simulink model "Rocket_Simulation"  (R2024a)
settings: Solver=VariableStepAuto  StartTime=0.0  StopTime=25  RelTol=1e-3
values from neighbouring files (symbols this model uses):
  g = -9.80665    [OpenRocketDataLoader.m]
undefined symbols (not defined in the file or in its folder): magnitude
libraries: simulink x3, aerolibactuator x1, aerolibatmos2 x1
settings Model: Creator=bennettbabu  LastModifiedBy=mason

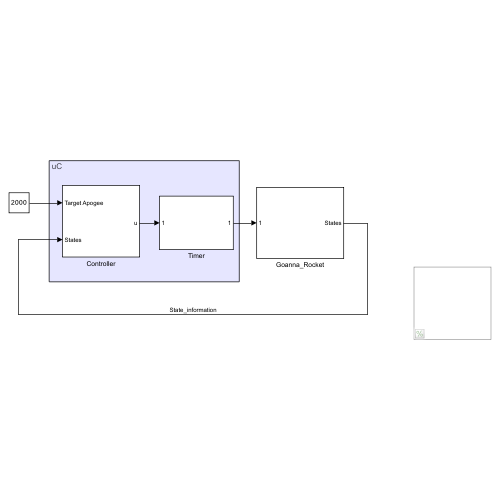
[thumbnail: Simulink's stored preview of the top-level diagram]
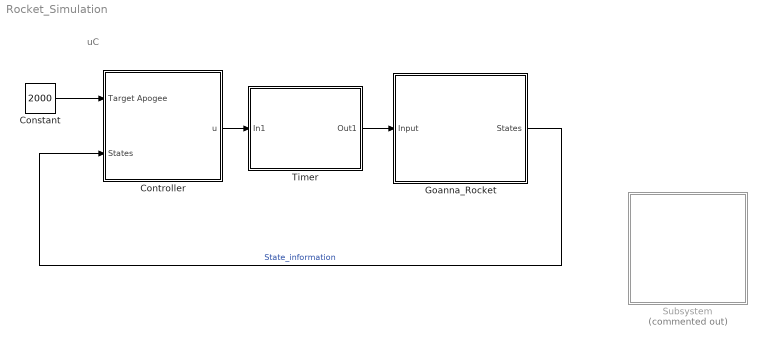
== system Rocket_Simulation ==
  note: uC
  Constant : Constant  Value=2000
  Controller : Subsystem
  Goanna_Rocket : Subsystem
  Subsystem : Subsystem  Commented=on
  Timer : Subsystem
  wires:
  Goanna_Rocket/1(States) -> Controller/2(States)  "State_information"
  Constant/1 -> Controller/1(Target Apogee)
  Controller/1(u) -> Timer/1(In1)
  Timer/1(Out1) -> Goanna_Rocket/1(Input)

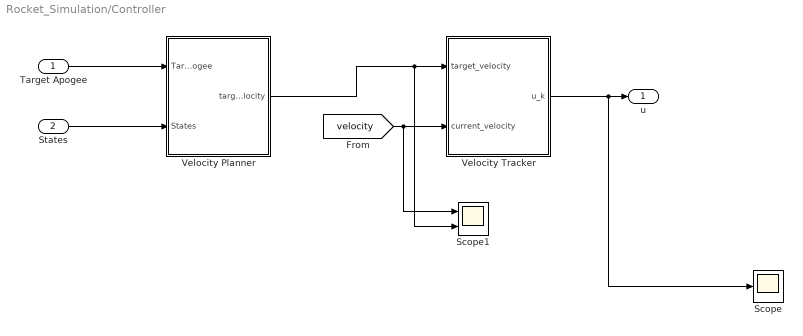
== system Rocket_Simulation/Controller ==
  Target Apogee : Inport
  States : Inport  Port=2
  Scope : Scope
  Scope1 : Scope  NumInputPorts=2
  Velocity Planner : Subsystem
  Velocity Tracker : Subsystem
  u : Outport
  wires:
  Target Apogee/1 -> Velocity Planner/1(Target Apogee)
  States/1 -> Velocity Planner/2(States)
  Velocity Tracker/1(u_k) -> Scope/1, u/1
  [velocity] -> Scope1/1, Velocity Tracker/2(current_velocity)
  Velocity Planner/1(target_velocity) -> Scope1/2, Velocity Tracker/1(target_velocity)

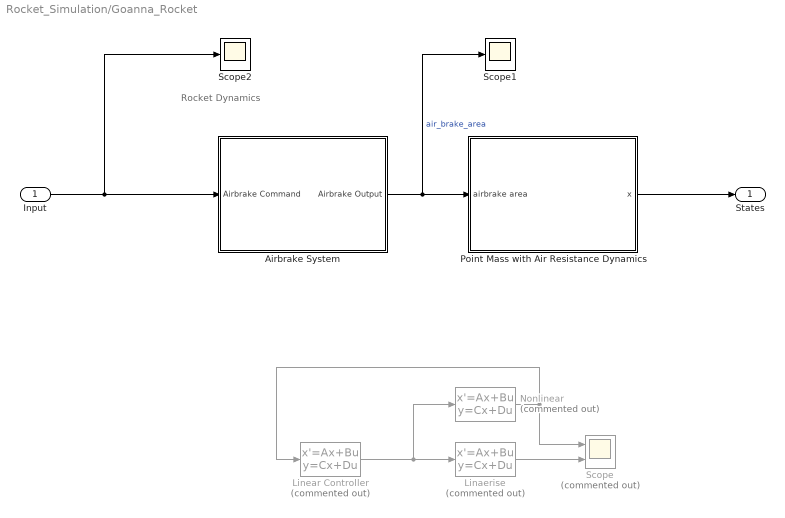
== system Rocket_Simulation/Goanna_Rocket ==
  note: Rocket Dynamics
  Input : Inport
  Airbrake System : Subsystem
      mask Display: image('airbrake.png');
  "Linaerise " : StateSpace  Commented=on  InitialCondition=0
  Linear Controller : StateSpace  Commented=on  InitialCondition=0
  Nonlinear : StateSpace  Commented=on  InitialCondition=0
  "Point Mass with Air Resistance Dynamics " : Subsystem
      mask Display: image('rocket.jpeg');
  Scope : Scope  Commented=on  NumInputPorts=2
  Scope1 : Scope
  Scope2 : Scope
  States : Outport
  wires:
  "Point Mass with Air Resistance Dynamics "/1(x) -> States/1
  Linear Controller/1 -> Nonlinear/1, "Linaerise "/1
  Nonlinear/1 -> Linear Controller/1, Scope/1
  "Linaerise "/1 -> Scope/2
  Input/1 -> Scope2/1, Airbrake System/1(Airbrake Command)
  Airbrake System/1(Airbrake Output) -> "Point Mass with Air Resistance Dynamics "/1(airbrake area), Scope1/1  "air_brake_area"

== system Rocket_Simulation/Subsystem ==
  wires:
  ? -> ?

== system Rocket_Simulation/Timer ==
  In1 : Inport
  Clock : Clock
  Constant1 : Constant  Value=0
  Switch : Switch  Criteria=u2 > Threshold  Threshold=5  SaturateOnIntegerOverflow=off  InputSameDT=off
  Out1 : Outport
  wires:
  Switch/1 -> Out1/1
  Clock/1 -> Switch/2
  In1/1 -> Switch/1
  Constant1/1 -> Switch/3

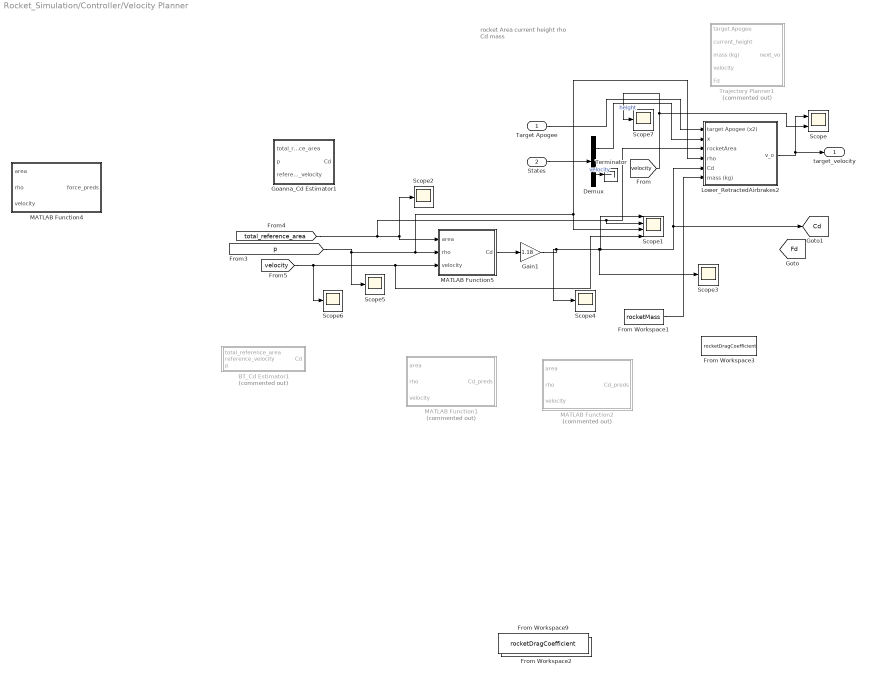
== system Rocket_Simulation/Controller/Velocity Planner ==
  note: rocket Area
      | current height
      | rho
      | Cd
      | mass
  Target Apogee : Inport
  States : Inport  Port=2
  BT_Cd Estimator1 : Subsystem  Commented=on
  Demux : Demux  Outputs=2
  From Workspace1 : FromWorkspace  VariableName=rocketMass
  From Workspace2 : FromWorkspace  VariableName=rocketDragCoefficient
  From Workspace3 : FromWorkspace  VariableName=rocketDragCoefficient
  From Workspace9 : FromWorkspace  VariableName=rocketDragCoefficient
  Gain1 : Gain  Gain=1.18
  Goanna_Cd Estimator1 : Subsystem
  Lower_RetractedAirbrakes2 : Subsystem
  MATLAB Function1 : MATLAB Function  Commented=on  TreatAsAtomicUnit=on
  MATLAB Function2 : MATLAB Function  Commented=on  TreatAsAtomicUnit=on
  MATLAB Function4 : MATLAB Function  TreatAsAtomicUnit=on
  MATLAB Function5 : MATLAB Function  TreatAsAtomicUnit=on
  Scope : Scope  NumInputPorts=2
  Scope1 : Scope  NumInputPorts=4
  Scope{2..7} (6 alike) : Scope
  Terminator : Terminator
  Trajectory Planner1 : Subsystem  Commented=on
  target_velocity : Outport
  tag scope: Cd=global, Fd=global
  wires:
  States/1 -> Demux/1
  Demux/1 -> Lower_RetractedAirbrakes2/2(x)  "height"
  Target Apogee/1 -> Lower_RetractedAirbrakes2/1(target Apogee (x2))
  [total_reference_area] -> Lower_RetractedAirbrakes2/3(rocketArea), Scope1/2, MATLAB Function5/1(area), Scope2/1
  Lower_RetractedAirbrakes2/1(v_o) -> Scope/1, target_velocity/1
  [velocity] -> MATLAB Function5/3(velocity), Scope1/4, Scope6/1
  [velocity] -> Scope/2, Scope7/1
  Gain1/1 -> Scope4/1, [Cd], Lower_RetractedAirbrakes2/5(Cd), Scope1/1, Scope3/1
  From Workspace1/1 -> Lower_RetractedAirbrakes2/6(mass (kg))
  [p] -> MATLAB Function5/2(rho), Lower_RetractedAirbrakes2/4(rho), Scope1/3, Scope5/1
  Demux/2 -> Terminator/1  "velocity"
  MATLAB Function5/1(Cd) -> Gain1/1

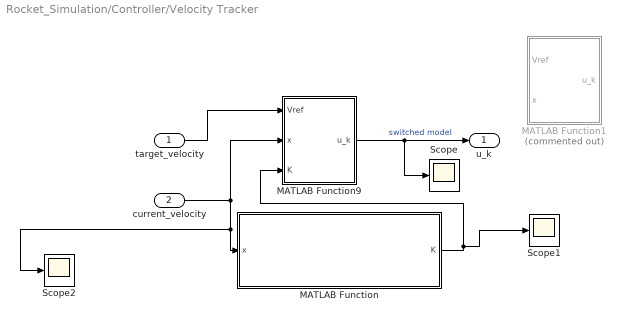
== system Rocket_Simulation/Controller/Velocity Tracker ==
  target_velocity : Inport
  current_velocity : Inport  Port=2
  MATLAB Function : MATLAB Function  TreatAsAtomicUnit=on
  MATLAB Function1 : MATLAB Function  Commented=on  TreatAsAtomicUnit=on
  MATLAB Function9 : MATLAB Function  TreatAsAtomicUnit=on
  Scope : Scope
  Scope1 : Scope
  Scope2 : Scope
  u_k : Outport
  wires:
  MATLAB Function9/1(u_k) -> Scope/1, u_k/1  "switched model"
  target_velocity/1 -> MATLAB Function9/1(Vref)
  MATLAB Function/1(K) -> Scope1/1, MATLAB Function9/3(K)
  current_velocity/1 -> Scope2/1, MATLAB Function/1(x), MATLAB Function9/2(x)

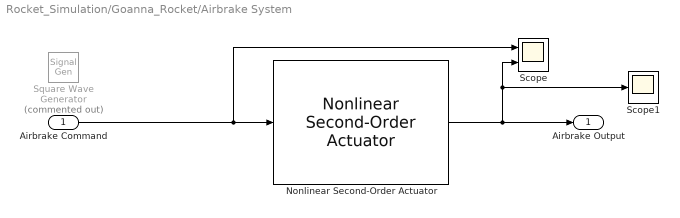
== system Rocket_Simulation/Goanna_Rocket/Airbrake System ==
  Airbrake Command : Inport
  Nonlinear Second-Order Actuator : aerolibactuator/Nonlinear Second-Order Actuator  wn_fin=10  z_fin=0.7  fin_max=maxAirbrakeArea  fin_min=0  fin_maxrate=315*pi/180  fin_act_0=0  fin_act_vel=0
  Scope : Scope  NumInputPorts=2
  Scope1 : Scope
  Square Wave Generator : SignalGenerator  Commented=on  WaveForm=square  Amplitude=0.01  Units=rad/sec
  Airbrake Output : Outport
  wires:
  Nonlinear Second-Order Actuator/1 -> Scope1/1, Scope/2, Airbrake Output/1
  Airbrake Command/1 -> Nonlinear Second-Order Actuator/1, Scope/1

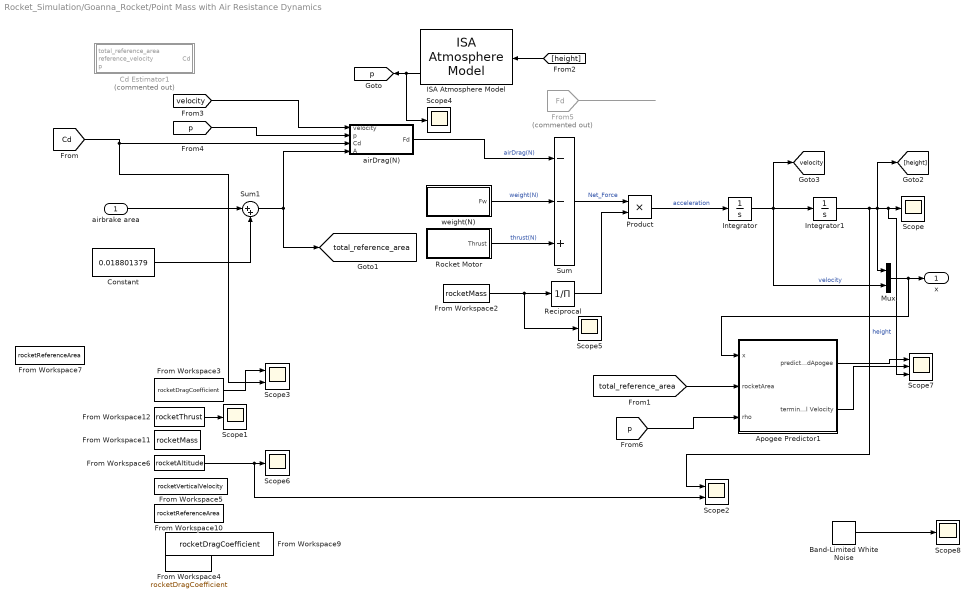
== system Rocket_Simulation/Goanna_Rocket/Point Mass with Air Resistance Dynamics  ==
  airbrake area : Inport
  Apogee Predictor1 : Subsystem
  Band-Limited White Noise : simulink/Sources/Band-Limited White Noise  Cov=[0.1]  Ts=0.1  seed=[23341]
  Cd Estimator1 : Subsystem  Commented=on
  Constant : Constant  Value=0.018801379
  From Workspace10 : FromWorkspace  VariableName=rocketReferenceArea
  From Workspace11 : FromWorkspace  VariableName=rocketMass
  From Workspace12 : FromWorkspace  VariableName=rocketThrust
  From Workspace2 : FromWorkspace  VariableName=rocketMass
  From Workspace3 : FromWorkspace  VariableName=rocketDragCoefficient
  From Workspace4 : FromWorkspace  VariableName=rocketDragCoefficient
  From Workspace5 : FromWorkspace  VariableName=rocketVerticalVelocity
  From Workspace6 : FromWorkspace  VariableName=rocketAltitude
  From Workspace7 : FromWorkspace  VariableName=rocketReferenceArea
  From Workspace9 : FromWorkspace  VariableName=rocketDragCoefficient
  From5 : From  Commented=on  GotoTag=Fd  TagVisibility=global
  ISA Atmosphere Model : aerolibatmos2/ISA Atmosphere Model  useExtended=off  action=Warning  custom=on  viscosityOut=off  g=9.80665  gamma=1.4  R=287.0531  L=0.0065  h_trop=11000  h_strat=20000  rho0=1.225  P0=101325  T0=288.15  h0=0  S=110.4  Tref=273.15  muref=1.716e-5
  Integrator : Integrator
  Integrator1 : Integrator
  Mux : Mux  Inputs=2
  Product : Product
  Reciprocal : Product  Inputs=/
  "Rocket Motor " : Subsystem
  Scope{,1,4..6,8} (6 alike) : Scope
  Scope2 : Scope  NumInputPorts=2
  Scope3 : Scope  NumInputPorts=2
  Scope7 : Scope  NumInputPorts=3
  Sum : Sum  Inputs=--+
  Sum1 : Sum  Inputs=|++
  airDrag(N) : Subsystem
  weight(N) : Subsystem
  x : Outport
  tag scope: p=global, total_reference_area=global, velocity=global
  wires:
  "Rocket Motor "/1(Thrust) -> Sum/3  "thrust(N)"
  weight(N)/1(Fw) -> Sum/2  "weight(N)"
  Sum/1 -> Product/1  "Net_Force"
  ISA Atmosphere Model/4 -> Scope4/1, [p]
  [height] -> ISA Atmosphere Model/1
  [velocity] -> airDrag(N)/1(velocity)
  [p] -> airDrag(N)/2(p)
  Product/1 -> Integrator/1  "acceleration"
  Integrator/1 -> [velocity], Integrator1/1, Mux/2  "velocity"
  Integrator1/1 -> Scope2/1, Mux/1, [height], Scope7/3, Scope/1  "height"
  Mux/1 -> Apogee Predictor1/1(x), x/1
  Reciprocal/1 -> Product/2
  From Workspace2/1 -> Scope5/1, Reciprocal/1
  From Workspace12/1 -> Scope1/1
  airbrake area/1 -> Sum1/1
  Sum1/1 -> [total_reference_area], airDrag(N)/4(A)
  Constant/1 -> Sum1/2
  [Cd] -> Scope3/2, airDrag(N)/3(Cd)
  From Workspace3/1 -> Scope3/1
  From5/1 -> ?
  airDrag(N)/1(Fd) -> Sum/1  "airDrag(N)"
  From Workspace6/1 -> Scope2/2, Scope6/1
  [total_reference_area] -> Apogee Predictor1/2(rocketArea)
  [p] -> Apogee Predictor1/3(rho)
  Apogee Predictor1/1(predictedApogee) -> Scope7/1
  Apogee Predictor1/2(terminal Velocity) -> Scope7/2
  Band-Limited White Noise/1 -> Scope8/1

== system Rocket_Simulation/Controller/Velocity Planner/BT_Cd Estimator1 ==
  total_reference_area : Inport
  reference_velocity : Inport  Port=2
  p : Inport  Port=3
  Rocket Specific Cd Estimator : MATLAB Function  TreatAsAtomicUnit=on
  Cd : Outport
  wires:
  Rocket Specific Cd Estimator/1(Cd) -> Cd/1
  total_reference_area/1 -> Rocket Specific Cd Estimator/1(SA)
  reference_velocity/1 -> Rocket Specific Cd Estimator/2(V)
  p/1 -> Rocket Specific Cd Estimator/3(rho)

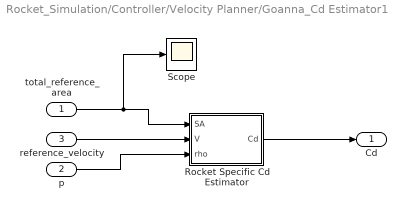
== system Rocket_Simulation/Controller/Velocity Planner/Goanna_Cd Estimator1 ==
  total_reference_area : Inport
  p : Inport  Port=2
  reference_velocity : Inport  Port=3
  Rocket Specific Cd Estimator : MATLAB Function  TreatAsAtomicUnit=on
  Scope : Scope
  Cd : Outport
  wires:
  Rocket Specific Cd Estimator/1(Cd) -> Cd/1
  total_reference_area/1 -> Scope/1, Rocket Specific Cd Estimator/1(SA)
  reference_velocity/1 -> Rocket Specific Cd Estimator/2(V)
  p/1 -> Rocket Specific Cd Estimator/3(rho)

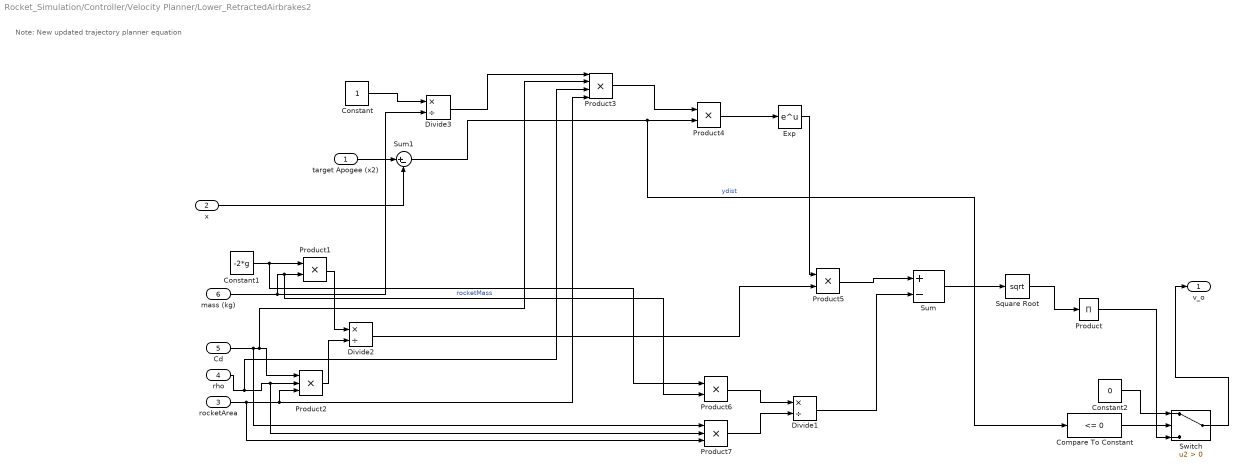
== system Rocket_Simulation/Controller/Velocity Planner/Lower_RetractedAirbrakes2 ==
  note: Note: New updated trajectory planner equation
  target Apogee (x2) : Inport
  x : Inport  Port=2
  rocketArea : Inport  Port=3
  rho : Inport  Port=4
  Cd : Inport  Port=5
  mass (kg) : Inport  Port=6
  Compare To Constant : simulink/Logic and Bit Operations/Compare To Constant  relop=<=  const=0  OutDataTypeStr=boolean
  Constant : Constant
  Constant1 : Constant  Value=-2*g
  Constant2 : Constant  Value=0
  Divide1 : Product  Inputs=*/
  Divide2 : Product  Inputs=*/
  Divide3 : Product  Inputs=*/
  Exp : Math
  Product : Product  Inputs=1
  Product{1,4..6} (4 alike) : Product
  Product2 : Product  Inputs=3
  Product3 : Product  Inputs=4
  Product7 : Product  Inputs=3
  Square Root : Sqrt
  Sum : Sum  Inputs=+-
  Sum1 : Sum  Inputs=|+-
  Switch : Switch  Criteria=u2 > Threshold  SaturateOnIntegerOverflow=off  InputSameDT=off
  v_o : Outport
  wires:
  target Apogee (x2)/1 -> Sum1/1
  Product2/1 -> Divide2/2
  Cd/1 -> Product7/1, Product3/2, Product2/1
  rocketArea/1 -> Product7/3, Product3/4, Product2/3
  Product1/1 -> Divide2/1
  Constant1/1 -> Product6/1, Product1/1
  rho/1 -> Product3/3, Product7/2, Product2/2
  mass (kg)/1 -> Divide3/2, Product6/2, Product1/2  "rocketMass"
  Divide3/1 -> Product3/1
  Product3/1 -> Product4/1
  Product4/1 -> Exp/1
  Divide2/1 -> Product5/2
  Exp/1 -> Product5/1
  Product5/1 -> Sum/1
  Divide1/1 -> Sum/2
  Product6/1 -> Divide1/1
  Product7/1 -> Divide1/2
  Sum/1 -> Square Root/1
  Constant/1 -> Divide3/1
  Switch/1 -> v_o/1
  Compare To Constant/1 -> Switch/2
  Sum1/1 -> Compare To Constant/1, Product4/2  "ydist"
  Constant2/1 -> Switch/1
  Square Root/1 -> Product/1
  Product/1 -> Switch/3
  x/1 -> Sum1/2

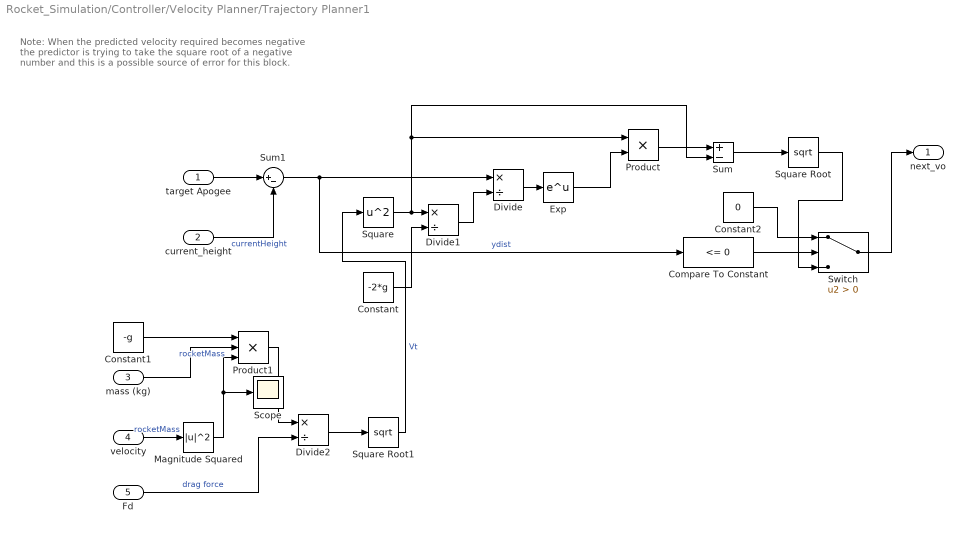
== system Rocket_Simulation/Controller/Velocity Planner/Trajectory Planner1 ==
  note: Note: When the predicted velocity required becomes negative the predictor is trying to take the square root of a negative number and this is a possible source of error for this block.
  target Apogee : Inport
  current_height : Inport  Port=2
  mass (kg) : Inport  Port=3
  velocity : Inport  Port=4
  Fd : Inport  Port=5
  Compare To Constant : simulink/Logic and Bit Operations/Compare To Constant  relop=<=  const=0  OutDataTypeStr=boolean
  Constant : Constant  Value=-2*g
  Constant1 : Constant  Value=-g
  Constant2 : Constant  Value=0
  Divide : Product  Inputs=*/
  Divide1 : Product  Inputs=*/
  Divide2 : Product  Inputs=*/
  Exp : Math
  Magnitude Squared : Math  Operator=magnitude^2
  Product : Product
  Product1 : Product  Inputs=3
  Scope : Scope
  Square : Math  Operator=square
  Square Root : Sqrt
  Square Root1 : Sqrt
  Sum : Sum  Inputs=+-
  Sum1 : Sum  Inputs=|+-
  Switch : Switch  Criteria=u2 > Threshold  SaturateOnIntegerOverflow=off  InputSameDT=off
  next_vo : Outport
  wires:
  Sum/1 -> Square Root/1
  Product/1 -> Sum/1
  Exp/1 -> Product/2
  Divide/1 -> Exp/1
  Sum1/1 -> Compare To Constant/1, Divide/1  "ydist"
  Constant/1 -> Divide1/2
  Divide1/1 -> Divide/2
  Square/1 -> Sum/2, Product/1, Divide1/1
  target Apogee/1 -> Sum1/1
  Square Root1/1 -> Square/1  "Vt"
  Divide2/1 -> Square Root1/1
  Product1/1 -> Divide2/1
  Constant1/1 -> Product1/1
  mass (kg)/1 -> Product1/2  "rocketMass"
  current_height/1 -> Sum1/2  "currentHeight"
  Compare To Constant/1 -> Switch/2
  Constant2/1 -> Switch/1
  Square Root/1 -> Switch/3
  Switch/1 -> next_vo/1
  Fd/1 -> Divide2/2  "drag force"
  velocity/1 -> Magnitude Squared/1  "rocketMass"
  Magnitude Squared/1 -> Product1/3, Scope/1

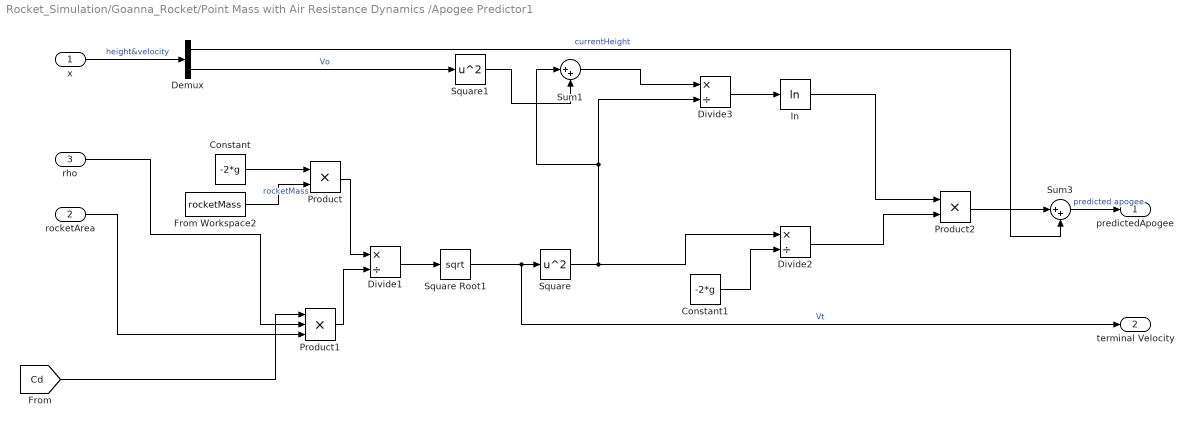
== system Rocket_Simulation/Goanna_Rocket/Point Mass with Air Resistance Dynamics /Apogee Predictor1 ==
  x : Inport
  rocketArea : Inport  Port=2
  rho : Inport  Port=3
  Constant : Constant  Value=-2*g
  Constant1 : Constant  Value=-2*g
  Demux : Demux  Outputs=2
  Divide1 : Product  Inputs=*/
  Divide2 : Product  Inputs=*/
  Divide3 : Product  Inputs=*/
  From Workspace2 : FromWorkspace  VariableName=rocketMass
  Product : Product
  Product1 : Product  Inputs=3
  Product2 : Product
  Square : Math  Operator=square
  Square Root1 : Sqrt
  Square1 : Math  Operator=square
  Sum1 : Sum  Inputs=|++
  Sum3 : Sum  Inputs=|++
  ln : Math  Operator=log
  predictedApogee : Outport
  terminal Velocity : Outport  Port=2
  wires:
  Constant/1 -> Product/1
  Product/1 -> Divide1/1
  Product1/1 -> Divide1/2
  [Cd] -> Product1/1
  rho/1 -> Product1/2
  rocketArea/1 -> Product1/3
  Divide1/1 -> Square Root1/1
  Square Root1/1 -> terminal Velocity/1, Square/1  "Vt"
  Product2/1 -> Sum3/1
  ln/1 -> Product2/1
  Divide2/1 -> Product2/2
  Square/1 -> Divide3/2, Sum1/1, Divide2/1
  Constant1/1 -> Divide2/2
  Divide3/1 -> ln/1
  Square1/1 -> Sum1/2
  Sum1/1 -> Divide3/1
  x/1 -> Demux/1  "height&velocity"
  From Workspace2/1 -> Product/2  "rocketMass"
  Demux/2 -> Square1/1  "Vo"
  Demux/1 -> Sum3/2  "currentHeight"
  Sum3/1 -> predictedApogee/1  "predicted apogee"

== system Rocket_Simulation/Goanna_Rocket/Point Mass with Air Resistance Dynamics /Cd Estimator1 ==
  total_reference_area : Inport
  reference_velocity : Inport  Port=2
  p : Inport  Port=3
  Rocket Specific Cd Estimator : MATLAB Function  TreatAsAtomicUnit=on
  Cd : Outport
  wires:
  Rocket Specific Cd Estimator/1(Cd) -> Cd/1
  total_reference_area/1 -> Rocket Specific Cd Estimator/1(SA)
  reference_velocity/1 -> Rocket Specific Cd Estimator/2(V)
  p/1 -> Rocket Specific Cd Estimator/3(rho)

== system Rocket_Simulation/Goanna_Rocket/Point Mass with Air Resistance Dynamics /Rocket Motor  ==
  From Workspace12 : FromWorkspace  VariableName=rocketThrust
  Gain : Gain  Gain=1.0
  Thrust : Outport
  wires:
  From Workspace12/1 -> Gain/1
  Gain/1 -> Thrust/1

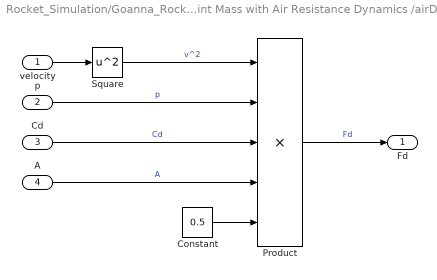
== system Rocket_Simulation/Goanna_Rocket/Point Mass with Air Resistance Dynamics /airDrag(N) ==
  velocity : Inport
  p : Inport  Port=2
  Cd : Inport  Port=3
  A : Inport  Port=4
  Constant : Constant  Value=0.5
  Product : Product  Inputs=5
  Square : Math  Operator=square
  Fd : Outport
  wires:
  velocity/1 -> Square/1
  Square/1 -> Product/1  "v^2"
  p/1 -> Product/2  "p"
  Cd/1 -> Product/3  "Cd"
  A/1 -> Product/4  "A"
  Constant/1 -> Product/5
  Product/1 -> Fd/1  "Fd"

== system Rocket_Simulation/Goanna_Rocket/Point Mass with Air Resistance Dynamics /weight(N) ==
  From Workspace11 : FromWorkspace  VariableName=rocketMass
  gravity : Gain  Gain=9.80665
  Fw : Outport
  wires:
  From Workspace11/1 -> gravity/1
  gravity/1 -> Fw/1

== matlab function Rocket_Simulation/Controller/Velocity Tracker/MATLAB Function9 ==
  data: Vref input; x input; u_k output; K input

function u_k = fcn(Vref, x,K)
     %% Measurements

    xref_k = Vref;
    x_k = x; % measured system states

     %uref_k = 8;
     u_k = -K * (x_k - xref_k);
    if u_k < 0
        u_k = 0;
    end
     return
end

== matlab function Rocket_Simulation/Controller/Velocity Planner/MATLAB Function1 ==
  data: area input; Cd_preds output; rho input; velocity input
function Cd_preds = predict_drag_coefficients(area, rho, velocity)
    % Load model parameters from the .mat file
    params = load('model_params.mat');
    area
    rho
    velocity = abs(velocity)
    % Generate predictions for a grid of velocities
    force_preds = arrayfun(@(v) poly_predict(area, rho, v, params), velocity);
    
    % Check if any of the inputs are zero
    if area ~= 0 && rho ~= 0 && all(velocity ~= 0)
        % Calculate Cd for each velocity

        Cd_preds = arrayfun(@(f, v) f / (0.5 * rho * area * v^2), force_preds, velocity)
        if Cd_preds <= 0
            Cd_preds = 0.386598;
        end 
    else
        % Assign default value if any input is zero
        Cd_preds = 0.386598;
    end
end

function y_pred = poly_predict(area, rho, velocity, params)
    % Extract the parameters
    scaler_X_mean = params.scaler_X_mean;
    scaler_X_std = params.scaler_X_std;
    scaler_y_mean = params.scaler_y_mean;
    scaler_y_std = params.scaler_y_std;
    coefficients = params.coefficients;
    intercept = params.intercept;

    % Standardize input features (This is required because the GPR was trained this way)
    X = [(area - scaler_X_mean(1)) / scaler_X_std(1), ...
         (rho - scaler_X_mean(2)) / scaler_X_std(2), ...
         (velocity - scaler_X_mean(3)) / scaler_X_std(3)];

    % Compute polynomial features up to the desired degree
    degree = 3;
    X_poly = get_poly_features(X, degree);

    % Predict using the polynomial model
    y_scaled = sum(coefficients .* X_poly) + intercept;

    % Inverse standardization of the prediction
    y_pred = y_scaled * scaler_y_std + scaler_y_mean;
end

function X_poly = get_poly_features(X, degree)
    % Generate polynomial features up to the desired degree
    n = length(X);
    X_poly = 1;  % constant bias term

    for d = 1:degree
        combos = nchoosek(repmat(1:n, 1, d), d);
        combos = unique(sort(combos, 2), 'rows');
        for i = 1:size(combos, 1)
            term = prod(X(combos(i, :)));
            X_poly = [X_poly, term];
        end
    end
end

== matlab function Rocket_Simulation/Controller/Velocity Planner/BT_Cd Estimator1/Rocket Specific Cd Estimator ==
  data: SA input; Cd output; V input; rho input
function Cd = fcn(SA,V,rho)
u1 =  43.32270126;  % Total rocket SA.
u2 = -0.000687709; % Velocity
u3 = 0.531869262; % Air density
intercept = -0.447146101;
Cd = (SA*u1)+ (V*u2)+ (rho*u3) + (intercept) ;
end

== matlab function Rocket_Simulation/Goanna_Rocket/Point Mass with Air Resistance Dynamics /Cd Estimator1/Rocket Specific Cd Estimator ==
  data: SA input; Cd output; V input; rho input
function Cd = fcn(SA,V,rho)
u1 =  43.32270126;  % Total rocket SA.
u2 = -0.000687709; % Velocity
u3 = 0.531869262; % Air density
intercept = -0.447146101;
Cd = (SA*u1)+ (V*u2)+ (rho*u3) + (intercept) ;
end

== matlab function Rocket_Simulation/Controller/Velocity Planner/Goanna_Cd Estimator1/Rocket Specific Cd Estimator ==
  data: SA input; Cd output; V input; rho input
function Cd = fcn(SA,V,rho)
u1 =  21.038140859140483;  % Total rocket SA.
u2 = -0.00013081819610389527; % Velocity
u3 = -0.01571134830357142; % Air density
intercept = -0.008812382900499849;
Cd = (SA*u1)+ (V*u2)+ (rho*u3) + (intercept) ;
end

== matlab function Rocket_Simulation/Controller/Velocity Planner/MATLAB Function2 ==
  data: area input; Cd_preds output; rho input; velocity input
function Cd_preds = predict_drag_coefficients(area, rho, velocity)
    % Load model parameters from the .mat file
    params = load('model_params.mat');
    velocity = abs(velocity); % Ensure velocities are positive
    
    % Generate predictions for a grid of velocities
    force_preds = arrayfun(@(v) poly_predict(area, rho, v, params), velocity);
    
    % Check if any of the inputs are zero
    if area ~= 0 && rho ~= 0 && all(velocity ~= 0)
        % Calculate Cd for each velocity
        Cd_preds = arrayfun(@(f, v) f / (0.5 * rho * area * v^2), force_preds, velocity);
        
        % Ensure all Cd_preds are positive
        Cd_preds(Cd_preds <= 0) = 0.386598;
    else
        % Assign default value if any input is zero
        Cd_preds = 0.386598 * ones(size(velocity));
    end
end

function y_pred = poly_predict(area, rho, velocity, params)
    % Extract the parameters
    scaler_X_mean = params.scaler_X_mean;
    scaler_X_std = params.scaler_X_std;
    scaler_y_mean = params.scaler_y_mean;
    scaler_y_std = params.scaler_y_std;
    coefficients = params.coefficients;
    intercept = params.intercept;

    % Standardize input features (This is required because the GPR was trained this way)
    X = [(area - scaler_X_mean(1)) / scaler_X_std(1), ...
         (rho - scaler_X_mean(2)) / scaler_X_std(2), ...
         (velocity - scaler_X_mean(3)) / scaler_X_std(3)];

    % Compute polynomial features up to the desired degree
    degree = 3;
    X_poly = get_poly_features(X, degree);

    % Predict using the polynomial model
    y_scaled = sum(coefficients .* X_poly) + intercept;

    % Inverse standardization of the prediction
    y_pred = y_scaled * scaler_y_std + scaler_y_mean;
end

function X_poly = get_poly_features(X, degree)
    % Generate polynomial features up to the desired degree
    n = length(X);
    X_poly = 1;  % constant bias term

    for d = 1:degree
        combos = nchoosek(repmat(1:n, 1, d), d);
        combos = unique(sort(combos, 2), 'rows');
        for i = 1:size(combos, 1)
            term = prod(X(combos(i, :)));
            X_poly = [X_poly, term];
        end
    end
end

== matlab function Rocket_Simulation/Controller/Velocity Planner/MATLAB Function5 ==
  data: area input; Cd output; rho input; velocity input
function Cd = cd_estimator(area, rho, velocity)
    % coefficients = [intercept, Area, Density, Velocity, Area^2, Area*Density, Area*Velocity, Density^2, Velocity^2];
    coefficients = [1.271359304570330, -89.2957223507969, -0.139915015095874, -0.000642306508177183, 2402.82168908320, 5.06245068661305, 0.0110556725929730, 0.00208924419408200, 6.72989011187282e-07];
    
    % Manually generate polynomial features for scalar inputs
    X_pred_poly = [1, ... % Intercept term
                   area, ... % Area
                   rho, ... % Density
                   velocity, ... % Velocity
                   area^2, ... % Area^2
                   area * rho, ... % Area * Density
                   area * velocity, ... % Area * Velocity
                   rho^2, ... % Density^2
                   velocity^2]; % Velocity^2
    
    Cd = X_pred_poly * coefficients';
end

== matlab function Rocket_Simulation/Controller/Velocity Planner/MATLAB Function4 ==
  data: area input; force_preds output; rho input; velocity input
function force_preds = predict_drag_coefficients(area, rho, velocity)
    area = abs(area);
    % Load model parameters from the .mat file
    params = load('force_pred.mat');
    velocity = abs(velocity); % Ensure velocities are positive

    if velocity >= 30
        % Generate predictions for a grid of velocities
        force_preds = arrayfun(@(v) poly_predict(area, rho, v, params), velocity);
    else
        force_preds = 0;
    end
   
    if force_preds < 0
        force_preds = 0.0;
    elseif isnan(force_preds)
        force_preds = 0.0;
    end

    if force_preds > 1000
        disp(force_preds)
        disp(area)
        disp(rho)
        disp(velocity)
    end
end

function y_pred = poly_predict(area, rho, velocity, params)
    % Extract the parameters
    scaler_X_mean = params.scaler_X_mean;
    scaler_X_std = params.scaler_X_std;
    scaler_y_mean = params.scaler_y_mean;
    scaler_y_std = params.scaler_y_std;
    coefficients = params.coefficients;
    intercept = params.intercept;

    % Standardize input features (This is required because the GPR was trained this way)
    X = [(area - scaler_X_mean(1)) / scaler_X_std(1), ...
         (rho - scaler_X_mean(2)) / scaler_X_std(2), ...
         (velocity - scaler_X_mean(3)) / scaler_X_std(3)];

    % Compute polynomial features up to the desired degree
    degree = 3;
    X_poly = get_poly_features(X, degree);

    % Predict using the polynomial model
    y_scaled = sum(coefficients .* X_poly) + intercept;

    % Inverse standardization of the prediction
    y_pred = y_scaled * scaler_y_std + scaler_y_mean;
end

function X_poly = get_poly_features(X, degree)
    % Generate polynomial features up to the desired degree
    n = length(X);
    X_poly = 1;  % constant bias term

    for d = 1:degree
        combos = nchoosek(repmat(1:n, 1, d), d);
        combos = unique(sort(combos, 2), 'rows');
        for i = 1:size(combos, 1)
            term = prod(X(combos(i, :)));
            X_poly = [X_poly, term];
        end
    end
end

== matlab function Rocket_Simulation/Controller/Velocity Tracker/MATLAB Function ==
  data: x input; K output
function K = GainSchedulingPolynomialAlgorithm(x)
%#codegen
%k = Gain 
%X =  rocket velocity

% Define the coefficients
a = -1e-5;
b = 0.0037;
c = -0.3743;

% Compute the quadratic equation
K = a*x^2 + b*x + c;

== matlab function Rocket_Simulation/Controller/Velocity Tracker/MATLAB Function1 ==
  data: Vref input; x input; u_k output

function u_k = fcn(Vref, x)
     %% Measurements

    xref_k = Vref;
    x_k = x; % measured system states
   %uref_k = 5;

    K = -0.035; %220m/s
    u_k = -K*(x_k-xref_k);
    if u_k < 0
        u_k = 0;
    end
    
    if (x<= 40)
     K =  -0.557604560965188;
     %uref_k = 8;
     u_k = -K * (x_k - xref_k)
    if u_k < 0
        u_k = 0;
    end
     return
   end 
    

   if (x<= 80)
     K =  -0.149050395144053;
     %uref_k = 10;
    u_k = -K * (x_k - xref_k)
    if u_k < 0
        u_k = 0;
    end
     return
   end 
    
   if (x <= 140)
    % uref_k = 13 ;
    K = -0.050007237207140;
    u_k = -K*(x_k-xref_k);
    if u_k < 0
        u_k = 0;
    end
    return
   end 

   if (x <= 180)
     %  uref_k = 15 ;
    K = -0.021944352703524;
    u_k = -K*(x_k-xref_k);
    if u_k < 0
        u_k = 0;
    end
    return

   end 
if u_k < 0
    u_k = 0;
end
end
